simulink model "LPT"  (R2025a)
settings: Solver=VariableStepAuto  StartTime=0.0  StopTime=10.0  RelTol=1e-3
undefined symbols (not defined in the file or in its folder): effMod_LPT, eta_lpt_map, PR_lpt_map, speed_vec_lpt, Wc_lpt_bp
settings Model: Creator=ramch  LastModifiedBy=ramch

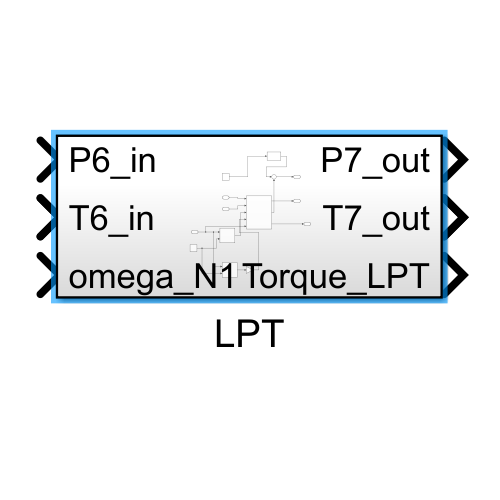
[thumbnail: Simulink's stored preview of the top-level diagram]
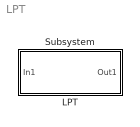
== system LPT ==
  LPT : Subsystem
  Subsystem : Subsystem

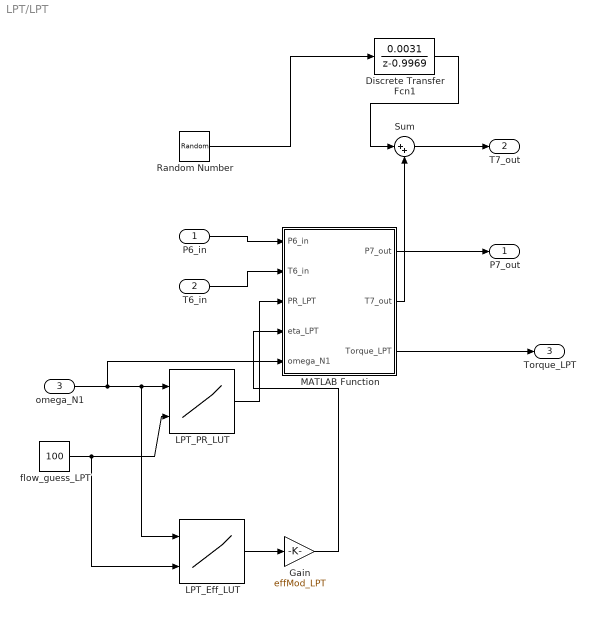
== system LPT/LPT ==
  P6_in : Inport
  T6_in : Inport  Port=2
  omega_N1 : Inport  Port=3
  Discrete Transfer Fcn1 : DiscreteTransferFcn  Numerator=0.0031  Denominator=1 -0.9969  InitialStates=0.001
  Gain : Gain  Gain=effMod_LPT
  LPT_Eff_LUT : Lookup_n-D  BreakpointsForDimension1=speed_vec_lpt  BreakpointsForDimension2=Wc_lpt_bp  Table=eta_lpt_map  InternalRulePriority=Speed  RndMeth=Simplest
      settings: InputPortMap=u0,u1
  LPT_PR_LUT : Lookup_n-D  BreakpointsForDimension1=speed_vec_lpt  BreakpointsForDimension2=Wc_lpt_bp  Table=PR_lpt_map  InternalRulePriority=Speed  RndMeth=Simplest
      settings: InputPortMap=u0,u1
  MATLAB Function : MATLAB Function  TreatAsAtomicUnit=on
  Random Number : RandomNumber  Variance=0.5  SampleTime=0.001
  Sum : Sum  Inputs=|++
  flow_guess_LPT : Constant  Value=100
  P7_out : Outport
  T7_out : Outport  Port=2
  Torque_LPT : Outport  Port=3
  wires:
  P6_in/1 -> MATLAB Function/1(P6_in)
  LPT_PR_LUT/1 -> MATLAB Function/3(PR_LPT)
  Random Number/1 -> Discrete Transfer Fcn1/1
  Discrete Transfer Fcn1/1 -> Sum/1
  Sum/1 -> T7_out/1
  T6_in/1 -> MATLAB Function/2(T6_in)
  omega_N1/1 -> MATLAB Function/5(omega_N1), LPT_Eff_LUT/1, LPT_PR_LUT/1
  flow_guess_LPT/1 -> LPT_PR_LUT/2, LPT_Eff_LUT/2
  MATLAB Function/3(Torque_LPT) -> Torque_LPT/1
  MATLAB Function/1(P7_out) -> P7_out/1
  LPT_Eff_LUT/1 -> Gain/1
  Gain/1 -> MATLAB Function/4(eta_LPT)
  MATLAB Function/2(T7_out) -> Sum/2

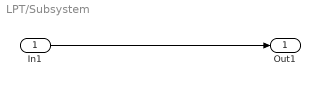
== system LPT/Subsystem ==
  In1 : Inport
  Out1 : Outport
  wires:
  In1/1 -> Out1/1

== matlab function LPT/MATLAB Function ==
  data: P6_in input; T6_in input; P7_out output; PR_LPT input; eta_LPT input; omega_N1 input; T7_out output; Torque_LPT output
function [P7_out, T7_out, Torque_LPT] = LPT_CalcCore(...
          P6_in, T6_in, PR_LPT, eta_LPT, omega_N1)
    gamma = 1.4;
    cp = 1004;
    P7_out = P6_in * PR_LPT;
    T7_out = T6_in * (1 - eta_LPT * (1 - PR_LPT^((gamma - 1)/gamma)));
    omega1 = omega_N1 * 2*pi/60;
    % Use placeholder flow of 100 kg/s (real flow from HPT later)
    m_dot_LPT = 100;  
    delta_h = cp * (T6_in - T7_out);
    Torque_LPT = (m_dot_LPT * delta_h) / omega1;
end
